simulink model "PID_Continuo"  (R2016a)
settings: Solver=ode45  StartTime=0.0  StopTime=10  MaxStep=1e-5  RelTol=1e-3
values from neighbouring files (symbols this model uses):
  K = 10    [actividad_2.m]
  Kd = K * c    [actividad_2.m]
  Ki = simplify(Ki)    [actividad_2.m]
  Kp = simplify(Kp)    [actividad_2.m]
  p1 = -3    [actividad_2.m]
  p2 = -2    [actividad_2.m]
  T = 0.09    [actividad_2.m]
settings Model: Creator=Usuario  LastModifiedBy=PC
settings DataIOCC: SaveFormat=Array  SignalLoggingSaveFormat=ModelDataLogs
settings OptimizationCC: InitFltsAndDblsToZero=on
settings DebuggingCC: SaveWithParameterizedLinksMsg=none  UnderspecifiedInitializationDetection=Classic  MergeDetectMultiDrivingBlocksExec=none  SignalResolutionControl=TryResolveAllWithWarning  SolverPrmCheckMsg=warning  MultiTaskDSMMsg=warning  MultiTaskCondExecSysMsg=none  FcnCallInpInsideContextMsg=UseLocalSettings
settings HardwareCC: ProdBitPerPointer=32  ProdLargestAtomicFloat=None  ProdIntDivRoundTo=Undefined  ProdEndianess=Unspecified  ProdWordSize=32  ProdHWDeviceType=32-bit Generic
settings ModelReferenceCC: PropagateSignalLabelsOutOfModel=off
settings GRTTargetCC: TargetFcnLib=ansi_tfl_tmw.mat  CombineOutputUpdateFcns=off  GRTInterface=on
settings ConfigComp: CovModelRefEnable=Off  CovSFcnEnable=off

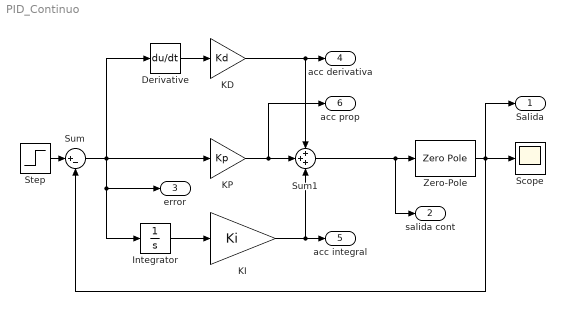
== system PID_Continuo ==
  Derivative : Derivative
  Integrator : Integrator
  KD : Gain  Gain=Kd
  KI : Gain  Gain=Ki
  KP : Gain  Gain=Kp
  Scope : Scope
  Step : Step  Time=0  SampleTime=T
  Sum : Sum  Inputs=|+-
  Sum1 : Sum  Inputs=+++
  Zero-Pole : ZeroPole  Zeros=[]  Poles=[p1 p2]  Gain=[K]
  Salida : Outport
  salida cont : Outport  Port=2
  error : Outport  Port=3
  acc derivativa : Outport  Port=4
  acc integral : Outport  Port=5
  acc prop : Outport  Port=6
  wires:
  Sum1/1 -> Zero-Pole/1, salida cont/1
  Step/1 -> Sum/1
  KI/1 -> Sum1/3, acc integral/1
  KP/1 -> acc prop/1, Sum1/2
  Zero-Pole/1 -> Sum/2, Scope/1, Salida/1
  Sum/1 -> Derivative/1, Integrator/1, error/1, KP/1
  KD/1 -> Sum1/1, acc derivativa/1
  Derivative/1 -> KD/1
  Integrator/1 -> KI/1
